simulink model "smc_metstoring"  (R2018b)
settings: Solver=FixedStepAuto  StartTime=0.0  StopTime=100.0  RelTol=1e-3
values from neighbouring files (symbols this model uses):
  xcos = 0:10    [variables.m]
  ycos = 0:10    [variables.m]
settings Model: Creator=axelwillekens  LastModifiedBy=axelwillekens

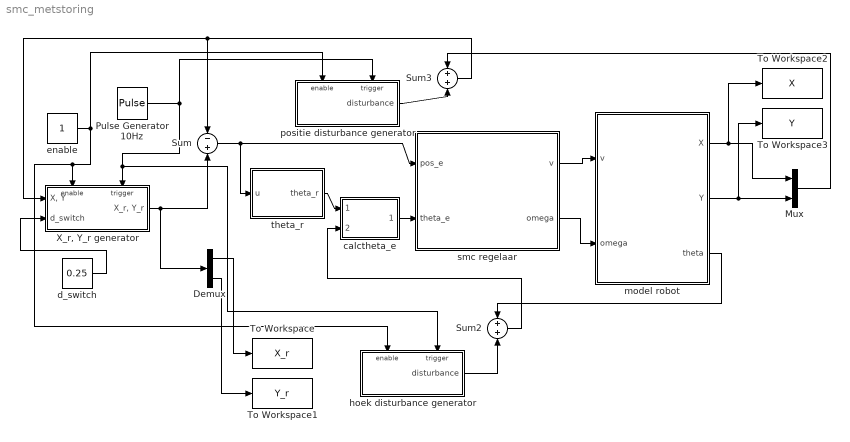
== system smc_metstoring ==
  Demux : Demux  Outputs=2
  Mux : Mux  Inputs=2
  Pulse Generator 10Hz : DiscretePulseGenerator  PulseType=Time based  Period=0.05  PulseWidth=5
  Sum : Sum  Inputs=-+
  Sum2 : Sum
  Sum3 : Sum
  To Workspace : ToWorkspace  VariableName=X_r  SaveFormat=Timeseries  SampleTime=-1
  To Workspace1 : ToWorkspace  VariableName=Y_r  SaveFormat=Timeseries  SampleTime=-1
  To Workspace2 : ToWorkspace  VariableName=X  SaveFormat=Timeseries  SampleTime=-1
  To Workspace3 : ToWorkspace  VariableName=Y  SaveFormat=Timeseries  SampleTime=-1
  "X_r, Y_r generator" : Subsystem  TreatAsAtomicUnit=on
  calctheta_e : MATLAB Function  TreatAsAtomicUnit=on
  d_switch : Constant  Value=0.25
  enable : Constant
  hoek disturbance generator : Subsystem  TreatAsAtomicUnit=on
  model robot : Subsystem
  positie disturbance generator : Subsystem  TreatAsAtomicUnit=on
  smc regelaar : MATLAB Function  TreatAsAtomicUnit=on
  theta_r : MATLAB Function  TreatAsAtomicUnit=on
  wires:
  "X_r, Y_r generator"/1("X_r, Y_r") -> Sum/2, Demux/1
  model robot/2(Y) -> To Workspace3/1, Mux/2
  model robot/1(X) -> To Workspace2/1, Mux/1
  Demux/1 -> To Workspace/1
  Demux/2 -> To Workspace1/1
  Mux/1 -> Sum3/1
  enable/1 -> positie disturbance generator/Enable, hoek disturbance generator/Enable, "X_r, Y_r generator"/Enable
  Pulse Generator 10Hz/1 -> hoek disturbance generator/Trigger, "X_r, Y_r generator"/Trigger, positie disturbance generator/Trigger
  Sum/1 -> theta_r/1(u), smc regelaar/1(pos_e)
  smc regelaar/2(omega) -> model robot/2(omega)
  smc regelaar/1(v) -> model robot/1(v)
  calctheta_e/1(theta_e) -> smc regelaar/2(theta_e)
  theta_r/1(theta_r) -> calctheta_e/1(theta_r)
  model robot/3(theta) -> Sum2/1
  d_switch/1 -> "X_r, Y_r generator"/2(d_switch)
  hoek disturbance generator/1(disturbance) -> Sum2/2
  Sum2/1 -> calctheta_e/2(theta)
  positie disturbance generator/1(disturbance) -> Sum3/2
  Sum3/1 -> Sum/1, "X_r, Y_r generator"/1("X, Y")

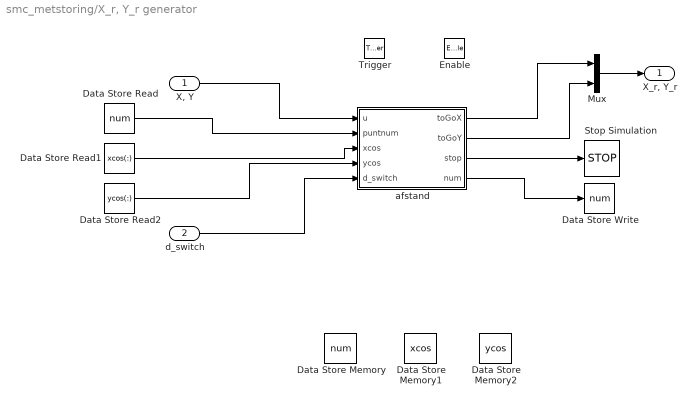
== system smc_metstoring/X_r, Y_r generator ==
  "X, Y" : Inport
  d_switch : Inport  Port=2
  Enable : EnablePort
  Trigger : TriggerPort  VariantControl=Variant
  Data Store Memory : DataStoreMemory  DataStoreName=num  ReadBeforeWriteMsg=warning  WriteAfterWriteMsg=warning  WriteAfterReadMsg=warning  InitialValue=1  ShowAdditionalParam=off
  Data Store Memory1 : DataStoreMemory  DataStoreName=xcos  ReadBeforeWriteMsg=warning  WriteAfterWriteMsg=warning  WriteAfterReadMsg=warning  InitialValue=linspace(0,30,101)  ShowAdditionalParam=off
  Data Store Memory2 : DataStoreMemory  DataStoreName=ycos  ReadBeforeWriteMsg=warning  WriteAfterWriteMsg=warning  WriteAfterReadMsg=warning  InitialValue=linspace(0,30,101)  ShowAdditionalParam=off
  Data Store Read : DataStoreRead  DataStoreName=num  DataStoreElements=num
  Data Store Read1 : DataStoreRead  DataStoreName=xcos  DataStoreElements=xcos(:)
  Data Store Read2 : DataStoreRead  DataStoreName=ycos  DataStoreElements=ycos(:)
  Data Store Write : DataStoreWrite  DataStoreName=num  DataStoreElements=num
  Mux : Mux  Inputs=2
  Stop Simulation : Stop
  afstand : MATLAB Function  TreatAsAtomicUnit=on
  "X_r, Y_r" : Outport
  wires:
  "X, Y"/1 -> afstand/1(u)
  afstand/1(toGoX) -> Mux/1
  afstand/3(stop) -> Stop Simulation/1
  Data Store Read/1 -> afstand/2(puntnum)
  afstand/4(num) -> Data Store Write/1
  Data Store Read1/1 -> afstand/3(xcos)
  Data Store Read2/1 -> afstand/4(ycos)
  afstand/2(toGoY) -> Mux/2
  Mux/1 -> "X_r, Y_r"/1
  d_switch/1 -> afstand/5(d_switch)

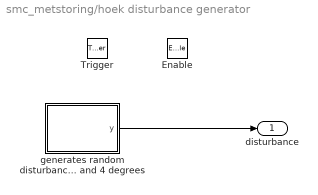
== system smc_metstoring/hoek disturbance generator ==
  Enable : EnablePort
  Trigger : TriggerPort  VariantControl=Variant
  generates random disturbance between -4 and 4 degrees : MATLAB Function  TreatAsAtomicUnit=on
  disturbance : Outport
  wires:
  generates random disturbance between -4 and 4 degrees/1(y) -> disturbance/1

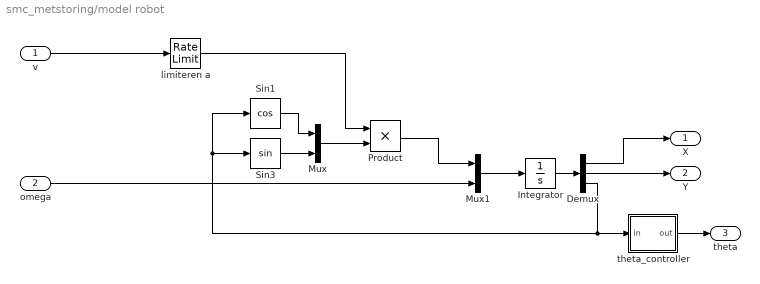
== system smc_metstoring/model robot ==
  v : Inport
  omega : Inport  Port=2
  Demux : Demux  Outputs=3
  Integrator : Integrator  InitialCondition=[0 0 -pi/4]
  Mux : Mux  Inputs=2
  Mux1 : Mux  Inputs=2
  Product : Product
  Sin1 : Trigonometry  Operator=cos
  Sin3 : Trigonometry
  limiteren a : RateLimiter  SampleTimeMode=inherited
  theta_controller : MATLAB Function  TreatAsAtomicUnit=on
  X : Outport
  Y : Outport  Port=2
  theta : Outport  Port=3
  wires:
  Sin1/1 -> Mux/1
  Sin3/1 -> Mux/2
  v/1 -> limiteren a/1
  limiteren a/1 -> Product/1
  Mux/1 -> Product/2
  Product/1 -> Mux1/1
  omega/1 -> Mux1/2
  Mux1/1 -> Integrator/1
  Integrator/1 -> Demux/1
  Demux/1 -> X/1
  Demux/2 -> Y/1
  Demux/3 -> Sin1/1, Sin3/1, theta_controller/1(in)
  theta_controller/1(out) -> theta/1

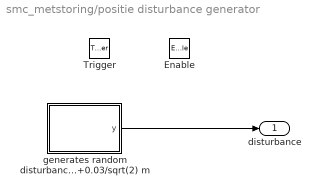
== system smc_metstoring/positie disturbance generator ==
  Enable : EnablePort
  Trigger : TriggerPort  VariantControl=Variant
  generates random disturbance between -0.03/sqrt(2) en +0.03/sqrt(2) m : MATLAB Function  TreatAsAtomicUnit=on
  disturbance : Outport
  wires:
  generates random disturbance between -0.03/sqrt(2) en +0.03/sqrt(2) m/1(y) -> disturbance/1

== matlab function smc_metstoring/X_r, Y_r generator/afstand ==
  data: u input; toGoX output; toGoY output; stop output; puntnum input; num output; xcos input; ycos input; d_switch input
function [toGoX, toGoY, stop, num] = fcn(u, puntnum, xcos, ycos, d_switch)
d = sqrt((xcos(puntnum)-u(1))^2 + (ycos(puntnum)-u(2))^2);
if d < d_switch
    num = puntnum + 1;
else
    num = puntnum;
end

toGoX = xcos(puntnum); 
toGoY = ycos(puntnum);

if num > length(xcos)
    stop = 1;
else
    stop = 0;
end

== matlab function smc_metstoring/smc regelaar ==
  data: pos_e input; v output; theta_e input; omega output
function [v,omega] = fcn(pos_e, theta_e)
v_r = 1;
omega_r = 0;
a_r = 0;
x_e = pos_e(1);
y_e = pos_e(2);
k2 = 0.2;
k1 = 0.4;
omega = omega_r + (y_e*a_r)/(1+(v_r*y_e)^2) + (v_r^2*sin(theta_e))/(1+(v_r*y_e)^2) + k2*min(1, max(-1, theta_e + atan(v_r*y_e)));
v = y_e*omega + v_r*cos(theta_e) + k1*min(1, max(-1,x_e));

== matlab function smc_metstoring/theta_r ==
  data: u input; theta_r output
function theta_r = fcn(u)

theta_r = atan2(u(2),u(1));

== matlab function smc_metstoring/hoek disturbance generator/generates random disturbance between -4 and 4 degrees ==
  data: y output
function y = fcn()
y = -4*(pi/180) + 2*4*(pi/180)*rand(1,1);

== matlab function smc_metstoring/positie disturbance generator/generates random disturbance between -0.03//sqrt(2) en +0.03//sqrt(2) m ==
  data: y output
function y = fcn()
y = [-0.03/sqrt(2) + 2*(0.03/sqrt(2))*rand(1,1),-0.03/sqrt(2) + 2*(0.03/sqrt(2))*rand(1,1)];

== matlab function smc_metstoring/model robot/theta_controller ==
  data: in input; out output
function out = fcn(in)

out = mod(in, 2*pi);

% nodig voor interval -180, +180
if out > pi
    out = out - 2*pi;
end

== matlab function smc_metstoring/calctheta_e ==
  data: theta_r input; theta_e output; theta input
function theta_e = fcn(theta_r,theta)
    
theta_e = theta_r - theta;

if theta_e > pi
    theta_e = theta_e - 2*pi;
elseif theta_e < -pi
    theta_e = theta_e + 2*pi;
end
